simulink model "lab10x2840x29_1"  (R2024a)
settings: Solver=VariableStepAuto  StartTime=0.0  StopTime=2
undefined symbols (not defined in the file): magnitude
libraries: dspstat3 x5, dspfdesign x2, dspsrcs4 x2, spspowerguiLib x1
settings Model: Creator=CS Net Games  LastModifiedBy=hp
settings SolverCC: AlgebraicLoopSolver=TrustRegion
settings DebuggingCC: UnconnectedInputMsg=warning  UnconnectedOutputMsg=warning  UnconnectedLineMsg=warning
settings ModelReferenceCC: EnableRefExpFcnMdlSchedulingChecks=on
settings SFSimCC: CustomCodeUndefinedFunction=UseInterfaceOnly
settings RTWCC: GPUComputeCapability=3.5

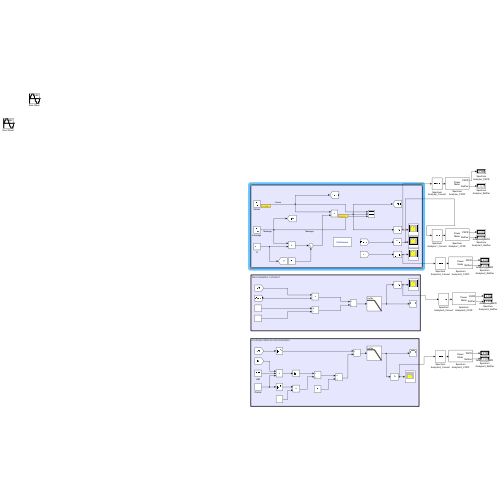
[thumbnail: Simulink's stored preview of the top-level diagram]
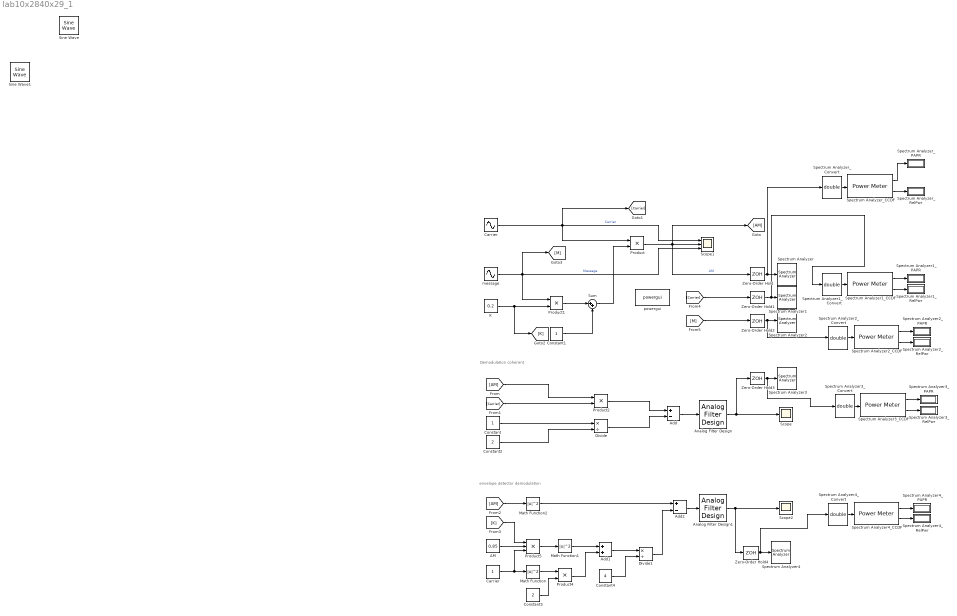
== system lab10x2840x29_1 ==
  note: envelope detector demodulation
  note: Demodulation coherent
  "AM " : Constant  Value=0.85
  Add : Sum  Inputs=+-
  Add1 : Sum
  Add2 : Sum  Inputs=+-
  Analog Filter Design : dspfdesign/Analog Filter Design  method=Butterworth  filttype=Lowpass  N=8  Wlo=pi*2*1500  Whi=80  Rp=2  Rs=40
  Analog Filter Design1 : dspfdesign/Analog Filter Design  method=Butterworth  filttype=Lowpass  N=10  Wlo=2*pi*1500  Whi=80  Rp=2  Rs=40
  Carrier : Sin  Frequency=pi*2*15000  SampleTime=0
  "Carrier " : Constant
  Constant : Constant
  Constant1 : Constant
  Constant2 : Constant  Value=2
  Constant3 : Constant  Value=2
  Constant4 : Constant  Value=4
  Divide : Product  Inputs=*/
  Divide1 : Product  Inputs=*/
  "K " : Constant  Value=0.2
  Math Function : Math  Operator=magnitude^2  SignedPower=on
  Math Function1 : Math  Operator=magnitude^2  SignedPower=on
  Math Function2 : Math  Operator=magnitude^2  SignedPower=on
  Product{,1..2,4} (4 alike) : Product
  Product5 : Product  Inputs=3
  Scope : Scope
  Scope1 : Scope  NumInputPorts=3
  Scope2 : Scope
  Sine Wave : dspsrcs4/Sine Wave  Amplitude=1  Frequency=15000  Phase=pi/2  SampleMode=Discrete  OutComplex=Real  CompMethod=Trigonometric fcn  TableSize=Speed  SampleTime=1/1000  SamplesPerFrame=1  ResetState=Restart at time zero  OutputFrames=off  dataType=double  wordLen=16  udDataType=sfix(16)  fracBitsMode=Best precision  numFracBits=15  OutDataTypeStr=double  LastOutDataTypeStr=double
  Sine Wave1 : dspsrcs4/Sine Wave  Amplitude=0.85  Frequency=1000  Phase=pi/2  SampleMode=Discrete  OutComplex=Real  CompMethod=Trigonometric fcn  TableSize=Speed  SampleTime=1/1000  SamplesPerFrame=1  ResetState=Restart at time zero  OutputFrames=off  dataType=double  wordLen=16  udDataType=sfix(16)  fracBitsMode=Best precision  numFracBits=15  OutDataTypeStr=double  LastOutDataTypeStr=double
  Spectrum Analyzer : SpectrumAnalyzer  WindowPosition=[0.000000,12.000000,1280.000000,697.000000,]  ScopeFrameLocation=window  SpectrumType=RMS  Method=Welch  SampleRate=150000  AxesScaling=Manual  AveragingMethod=Running  SpectrumUnits=Vrms  YLimits=[-0.07839420767346499952,0.70554787523022177709]  AllowFFTLengthLessThanSamplesPerUpdate=on  DefaultConfigurationName=spbscopes.SpectrumAnalyzerBlockCfg  IsFrequencyInputMode=0  FrequencyVectorPort=0  FrequencyVectorFromPort=0  FrequencyInputRBWPort=0  FrequencyInputRBWFromPort=0
      settings: OpenAtSimulationStart=off
  Spectrum Analyzer1 : SpectrumAnalyzer  WindowPosition=[0.000000,12.000000,1280.000000,697.000000,]  ScopeFrameLocation=window  SpectrumType=RMS  Method=Welch  SampleRate=150000  AxesScaling=Manual  AveragingMethod=Running  SpectrumUnits=Vrms  YLimits=[-0.056311512071834490811,0.50680361749574887043]  SelectedToolstripTab=spectrumAnalyzerToolstrip.measurementsTab  AllowFFTLengthLessThanSamplesPerUpdate=on  DefaultConfigurationName=spbscopes.SpectrumAnalyzerBlockCfg  IsFrequencyInputMode=0  FrequencyVectorPort=0  FrequencyVectorFromPort=0  FrequencyInputRBWPort=0  FrequencyInputRBWFromPort=0
      settings: OpenAtSimulationStart=off
  Spectrum Analyzer1_CCDF : dspstat3/Power Meter  Measurement=Peak-to-average power ratio  ReferenceLoad=1  OutputPowerUnits=dBm  WindowLength=256  OverlapLength=255  AllowArbitraryInputLength=off  ComputeCCDF=on  PowerRange=50  PowerResolution=0.1  CCDFOutput=Relative power (dB above average power)  ProbabilityVector=[ 10; 1; 0.1; 0.01; 0.001; 0.0001 ]  RelativePowerVector=[ 0; 3; 6; 9; 12 ]  ResetPort=off  SimulateUsing=Interpreted execution
  Spectrum Analyzer1_Convert : DataTypeConversion  OutDataTypeStr=double
  Spectrum Analyzer1_PAPR : Display
  Spectrum Analyzer1_RelPwr : Display
  Spectrum Analyzer2 : SpectrumAnalyzer  WindowPosition=[0.000000,12.000000,1280.000000,697.000000,]  ScopeFrameLocation=window  SpectrumType=RMS  Method=Welch  AxesScaling=Manual  AveragingMethod=Running  SpectrumUnits=Vrms  YLimits=[-0.047864785114428973212,0.43078307242832725166]  AllowFFTLengthLessThanSamplesPerUpdate=on  DefaultConfigurationName=spbscopes.SpectrumAnalyzerBlockCfg  IsFrequencyInputMode=0  FrequencyVectorPort=0  FrequencyVectorFromPort=0  FrequencyInputRBWPort=0  FrequencyInputRBWFromPort=0
      settings: OpenAtSimulationStart=off
  Spectrum Analyzer2_CCDF : dspstat3/Power Meter  Measurement=Peak-to-average power ratio  ReferenceLoad=1  OutputPowerUnits=dBm  WindowLength=256  OverlapLength=255  AllowArbitraryInputLength=off  ComputeCCDF=on  PowerRange=50  PowerResolution=0.1  CCDFOutput=Relative power (dB above average power)  ProbabilityVector=[ 10; 1; 0.1; 0.01; 0.001; 0.0001 ]  RelativePowerVector=[ 0; 3; 6; 9; 12 ]  ResetPort=off  SimulateUsing=Interpreted execution
  Spectrum Analyzer2_Convert : DataTypeConversion  OutDataTypeStr=double
  Spectrum Analyzer2_PAPR : Display
  Spectrum Analyzer2_RelPwr : Display
  Spectrum Analyzer3 : SpectrumAnalyzer  WindowPosition=[1.000000,1.000000,1280.000000,697.000000,]  ScopeFrameLocation=window  SpectrumType=RMS  Method=Welch  SampleRate=150000  AxesScaling=Manual  AveragingMethod=Running  SpectrumUnits=Vrms  YLimits=[-0.6909096549460655,1.2100077452440468]  AllowFFTLengthLessThanSamplesPerUpdate=on  DefaultConfigurationName=spbscopes.SpectrumAnalyzerBlockCfg  IsFrequencyInputMode=0  FrequencyVectorPort=0  FrequencyVectorFromPort=0  FrequencyInputRBWPort=0  FrequencyInputRBWFromPort=0
  Spectrum Analyzer3_CCDF : dspstat3/Power Meter  Measurement=Peak-to-average power ratio  ReferenceLoad=1  OutputPowerUnits=dBm  WindowLength=256  OverlapLength=255  AllowArbitraryInputLength=off  ComputeCCDF=on  PowerRange=50  PowerResolution=0.1  CCDFOutput=Relative power (dB above average power)  ProbabilityVector=[ 10; 1; 0.1; 0.01; 0.001; 0.0001 ]  RelativePowerVector=[ 0; 3; 6; 9; 12 ]  ResetPort=off  SimulateUsing=Interpreted execution
  Spectrum Analyzer3_Convert : DataTypeConversion  OutDataTypeStr=double
  Spectrum Analyzer3_PAPR : Display
  Spectrum Analyzer3_RelPwr : Display
  Spectrum Analyzer4 : SpectrumAnalyzer  WindowPosition=[1.000000,1.000000,1280.000000,697.000000,]  ScopeFrameLocation=window  SpectrumType=RMS  Method=Welch  SampleRate=150000  AxesScaling=Manual  AveragingMethod=Running  SpectrumUnits=Vrms  YLimits=[-0.15352407908271434311,1.3817167119597739688]  AllowFFTLengthLessThanSamplesPerUpdate=on  DefaultConfigurationName=spbscopes.SpectrumAnalyzerBlockCfg  IsFrequencyInputMode=0  FrequencyVectorPort=0  FrequencyVectorFromPort=0  FrequencyInputRBWPort=0  FrequencyInputRBWFromPort=0
      settings: OpenAtSimulationStart=off
  Spectrum Analyzer4_CCDF : dspstat3/Power Meter  Measurement=Peak-to-average power ratio  ReferenceLoad=1  OutputPowerUnits=dBm  WindowLength=256  OverlapLength=255  AllowArbitraryInputLength=off  ComputeCCDF=on  PowerRange=50  PowerResolution=0.1  CCDFOutput=Relative power (dB above average power)  ProbabilityVector=[ 10; 1; 0.1; 0.01; 0.001; 0.0001 ]  RelativePowerVector=[ 0; 3; 6; 9; 12 ]  ResetPort=off  SimulateUsing=Interpreted execution
  Spectrum Analyzer4_Convert : DataTypeConversion  OutDataTypeStr=double
  Spectrum Analyzer4_PAPR : Display
  Spectrum Analyzer4_RelPwr : Display
  Spectrum Analyzer_CCDF : dspstat3/Power Meter  Measurement=Peak-to-average power ratio  ReferenceLoad=1  OutputPowerUnits=dBm  WindowLength=256  OverlapLength=255  AllowArbitraryInputLength=off  ComputeCCDF=on  PowerRange=50  PowerResolution=0.1  CCDFOutput=Relative power (dB above average power)  ProbabilityVector=[ 10; 1; 0.1; 0.01; 0.001; 0.0001 ]  RelativePowerVector=[ 0; 3; 6; 9; 12 ]  ResetPort=off  SimulateUsing=Interpreted execution
  Spectrum Analyzer_Convert : DataTypeConversion  OutDataTypeStr=double
  Spectrum Analyzer_PAPR : Display
  Spectrum Analyzer_RelPwr : Display
  Sum : Sum  Inputs=|++
  Zero-Order Hold : ZeroOrderHold  SampleTime=1/(10*15e3)
  Zero-Order Hold1 : ZeroOrderHold  SampleTime=1/(10*15e3)
  Zero-Order Hold2 : ZeroOrderHold  SampleTime=1/(10*1e3)
  Zero-Order Hold3 : ZeroOrderHold  SampleTime=-1
  Zero-Order Hold4 : ZeroOrderHold  SampleTime=-1
  "message " : Sin  Amplitude=0.85  Frequency=pi*2*1000  SampleTime=0
  powergui : spspowerguiLib/powergui  Priority=1  SimulationMode=Continuous  SampleTime=50e-6  frequency=60  Iterations=50  frequencyindice=60  Pbase=100e6  ErrMax=1e-4  UnitsV=kV  UnitsW=MW  buscounter=0  FunctionMessages=off  echomessages=off  EnableUseOfTLC=off  CurrentSourceSwitches=off  DisableSnubberDevices=off  DisableRonSwitches=off  DisableVfSwitches=off  DisplayEquations=off  AutomaticDiscreteSolvers=off  SolverType=Tustin/Backward Euler (TBE)  Interpol=off  ExternalGateDelay=off  methode=off  Ts=100  x0status=blocks  SPID=on  SwTol=0  HookPort=off  NonlinearTolerance=0  nMaxIteration=15  ContinueOnMaxIteration=off  RestoreLinks=warning  ResistiveCurrentMeasurement=off  Frange=[0:2:500]  Ylog=off  Xlog=on  ShowGrid=off  save=off  variable=ZData  structure=0  ZoomFFT=off  StartTime=0.0  cycles=1  DisplayStyle=1  fundamental=60  FreqAxis=off  MaxFrequency=1000  frequencyindicesteady=1  RmsSteady=1  display=off
  wires:
  Zero-Order Hold1/1 -> Spectrum Analyzer1/1, Spectrum Analyzer1_Convert/1
  Zero-Order Hold2/1 -> Spectrum Analyzer2/1, Spectrum Analyzer2_Convert/1
  [M] -> Zero-Order Hold2/1
  "message "/1 -> Scope1/3, Product1/1, [M]  "Message"
  "K "/1 -> [K], Product1/2
  Sum/1 -> Product/2
  Product1/1 -> Sum/1
  Carrier/1 -> Scope1/1, Product/1, [Carrier]  "Carrier"
  Zero-Order Hold/1 -> Spectrum Analyzer/1, Spectrum Analyzer_Convert/1
  Constant1/1 -> Sum/2
  [Carrier] -> Zero-Order Hold1/1
  Product/1 -> Zero-Order Hold/1, [AM], Scope1/2  "AM"
  [Carrier] -> Product2/2
  Constant2/1 -> Divide/2
  Add/1 -> Analog Filter Design/1
  Analog Filter Design/1 -> Scope/1, Zero-Order Hold3/1
  Divide/1 -> Add/2
  [AM] -> Product2/1
  Constant/1 -> Divide/1
  Product2/1 -> Add/1
  Math Function/1 -> Product4/1
  "AM "/1 -> Product5/2
  Add2/1 -> Analog Filter Design1/1
  Analog Filter Design1/1 -> Zero-Order Hold4/1, Scope2/1
  Math Function2/1 -> Add2/1
  [AM] -> Math Function2/1
  Product4/1 -> Add1/2
  Divide1/1 -> Add2/2
  Product5/1 -> Math Function1/1
  Math Function1/1 -> Add1/1
  Constant4/1 -> Divide1/2
  "Carrier "/1 -> Math Function/1, Product5/3
  Constant3/1 -> Product4/2
  [K] -> Product5/1
  Add1/1 -> Divide1/1
  Zero-Order Hold3/1 -> Spectrum Analyzer3/1, Spectrum Analyzer3_Convert/1
  Zero-Order Hold4/1 -> Spectrum Analyzer4/1, Spectrum Analyzer4_Convert/1
  Spectrum Analyzer4_Convert/1 -> Spectrum Analyzer4_CCDF/1
  Spectrum Analyzer4_CCDF/1 -> Spectrum Analyzer4_PAPR/1
  Spectrum Analyzer4_CCDF/2 -> Spectrum Analyzer4_RelPwr/1
  Spectrum Analyzer3_Convert/1 -> Spectrum Analyzer3_CCDF/1
  Spectrum Analyzer3_CCDF/1 -> Spectrum Analyzer3_PAPR/1
  Spectrum Analyzer3_CCDF/2 -> Spectrum Analyzer3_RelPwr/1
  Spectrum Analyzer2_Convert/1 -> Spectrum Analyzer2_CCDF/1
  Spectrum Analyzer2_CCDF/1 -> Spectrum Analyzer2_PAPR/1
  Spectrum Analyzer2_CCDF/2 -> Spectrum Analyzer2_RelPwr/1
  Spectrum Analyzer1_Convert/1 -> Spectrum Analyzer1_CCDF/1
  Spectrum Analyzer1_CCDF/1 -> Spectrum Analyzer1_PAPR/1
  Spectrum Analyzer1_CCDF/2 -> Spectrum Analyzer1_RelPwr/1
  Spectrum Analyzer_Convert/1 -> Spectrum Analyzer_CCDF/1
  Spectrum Analyzer_CCDF/1 -> Spectrum Analyzer_PAPR/1
  Spectrum Analyzer_CCDF/2 -> Spectrum Analyzer_RelPwr/1
